simulink model "Citation"  (Simulink 10.1)
settings: Solver=ode5  StartTime=0.0  StopTime=100  FixedStep=0.01  RelTol=1e-3  EnableMultiTasking=on
values from neighbouring files (symbols this model uses):
  cv1 = 20000    [gear_params.m]
  cv2 = cv1    (= 20000)    [gear_params.m]
  cv3 = 4000    [gear_params.m]
  cv4 = 20000    [gear_params.m]
  deltagmax1 = 0.25    [gear_params.m]
  deltagmax2 = deltagmax1    (= 0.25)    [gear_params.m]
  deltagmax3 = 0.24    [gear_params.m]
  deltagmax4 = 0.02    [gear_params.m]
  kt1 = 525020    [gear_params.m]
  kt2 = kt1    (= 525020)    [gear_params.m]
  kt3 = 457050    [gear_params.m]
  murol = 0.03*10    (= 0.3)    [gear_params.m]
  P1 = 2000    [gear_params.m]
  P2 = P1    (= 2000)    [gear_params.m]
  P3 = 2550    [gear_params.m]
  P4 = 40000    [gear_params.m]
  x0 = []    [cessnac550_3d_sfnc.m]    (also in sfunxyz.m)
  xl1 = xcg-6.858    [gear_params.m]
  xl2 = xcg-6.858    [gear_params.m]
  xl3 = xcg-2.0752    [gear_params.m]
  xl4 = xcg-12.742    [gear_params.m]
  yl1 = 1.918    [gear_params.m]
  yl2 = -1.918    [gear_params.m]
  yl3 = 0    [gear_params.m]
  yl4 = 0    [gear_params.m]
  zl1 = zcg-1.701    [gear_params.m]
  zl2 = zcg-1.701    [gear_params.m]
  zl3 = zcg-1.7488    [gear_params.m]
  zl4 = zcg-2.78    [gear_params.m]
undefined symbols (not defined in the file or in its folder): chord, Deng, ealphag, ealphas, g0, hDME, hGS, lh, massinit, matbuaf, matdaf, matdam, matdbbf, matdeaf, matdgaf, matdqaf, matduaf, matdwaw, matedhr, mateif, matelhr, matemhr, matemv1, matemv2, matemve, matetam, mateuaf, matfaaf, matfaxl, matff, matibaf, matibmh, matipaf, matipmh, matiraf, matiuaf, matiwaf, matlaf, matlam, matleaf, matleam, matlgaf, matlqaf, matluaf, matmaaf, matmaam, matmaf, matmam, matmbbf, matmeaf, matmeam, matmgaf, matmqaf, matmrbr, matn1d, matn2d, matnbab, matnbaf, matnbmh, matnpaf ... (+49)
undefined symbols (not defined in the file): matibb
libraries: vrlib x1
(part 4 of 4)

== system Citation/Cessna Citation 500/Citation model DASMAT/AIRCRAFT MODEL/AFM/Aeromod/SubSystem/model/CLCAL/CLGEAF ==
  alpha : Inport
  deltaf : Inport  Port=2
  Prod : Product  InputSameDT=on  SaturateOnIntegerOverflow=on  OutDataTypeStr=Inherit: Same as first input
  Sat : Saturate  UpperLimit=0.04  LowerLimit=-inf
  Sum : Sum  InputSameDT=on  SaturateOnIntegerOverflow=on  OutDataTypeStr=Inherit: Same as first input
  VDOMMYR37 : Lookup  InputValues=vdommyr37(1,:)  Table=vdommyr37(2,:)  SaturateOnIntegerOverflow=on
  VDOMMYR40 : Gain  Gain=1.6  SaturateOnIntegerOverflow=on  OutDataTypeStr=Inherit: Same as input  ParamDataTypeStr=Inherit: Same as input
  rad2deg : Gain  Gain=(180/pi)  SaturateOnIntegerOverflow=on  OutDataTypeStr=Inherit: Same as input  ParamDataTypeStr=Inherit: Same as input
  CLGEAF : Outport
  wires:
  VDOMMYR37/1 -> VDOMMYR40/1, Prod/2
  rad2deg/1 -> Prod/1
  Sat/1 -> rad2deg/1
  alpha/1 -> Sat/1
  deltaf/1 -> VDOMMYR37/1
  VDOMMYR40/1 -> Sum/2
  Prod/1 -> Sum/1
  Sum/1 -> CLGEAF/1

== system Citation/Cessna Citation 500/Citation model DASMAT/AIRCRAFT MODEL/AFM/Aeromod/SubSystem/model/CLCAL/SP0 ==
  deltae : Inport
  Abs : Abs  SaturateOnIntegerOverflow=on
  Fcn : Fcn  Expr=(0.087+0.25*(u[1]-0.087))/(u[1]+1e-11)
  Prod : Product  InputSameDT=on  SaturateOnIntegerOverflow=on  OutDataTypeStr=Inherit: Same as first input
  Sat : Saturate  UpperLimit=1  LowerLimit=-inf
  SP0 : Outport
  wires:
  deltae/1 -> Prod/1, Abs/1
  Sat/1 -> Prod/2
  Fcn/1 -> Sat/1
  Abs/1 -> Fcn/1
  Prod/1 -> SP0/1

== system Citation/Cessna Citation 500/Citation model DASMAT/AIRCRAFT MODEL/AFM/Aeromod/SubSystem/model/CLLCAL/CIBAB ==
  note: 02-11-2000
      | Modified by A. R. Veldhuijzen
      | sftable3.m was replaced with table3.dll
      | X and Y are exchanged in this Mathworks implementation
  x0 : Inport
  y0 : Inport  Port=2
  z0 : Inport  Port=3
  Mux : Mux  Inputs=3
  S-function : S-Function  FunctionName=table3  Parameters=yindex, xindex ,zindex, table  SFunctionDeploymentMode=off  EnableBusSupport=off
  out_1 : Outport
  wires:
  z0/1 -> Mux/3
  y0/1 -> Mux/1
  x0/1 -> Mux/2
  Mux/1 -> S-function/1
  S-function/1 -> out_1/1

== system Citation/Cessna Citation 500/Citation model DASMAT/AIRCRAFT MODEL/AFM/Aeromod/SubSystem/model/CLLCAL/LFACT ==
  hcg : Inport
  Sat : Saturate  UpperLimit=1  LowerLimit=0
  hrunway : Fcn  Expr=1-(u[1]-1)/30
  LFACT : Outport
  wires:
  Sat/1 -> LFACT/1
  hcg/1 -> hrunway/1
  hrunway/1 -> Sat/1

== system Citation/Cessna Citation 500/Citation model DASMAT/AIRCRAFT MODEL/AFM/Aeromod/SubSystem/model/CMCAL/EALPHA ==
  alpha : Inport
  deltaf : Inport  Port=2
  Fcn : Fcn  Expr=1-u[1]*u[2]
  Mux : Mux  Inputs=2
  Sat : Saturate  UpperLimit=1  LowerLimit=0
  Sum : Sum  Inputs=+-  InputSameDT=on  SaturateOnIntegerOverflow=on  OutDataTypeStr=Inherit: Same as first input
  ealphag : Lookup  InputValues=ealphag(1,:)  Table=ealphag(2,:)  SaturateOnIntegerOverflow=on
  ealphas : Lookup  InputValues=ealphas(1,:)  Table=ealphas(2,:)  SaturateOnIntegerOverflow=on
  EALPHA : Outport
  wires:
  deltaf/1 -> ealphag/1, ealphas/1
  alpha/1 -> Sum/1
  Mux/1 -> Fcn/1
  ealphag/1 -> Mux/2
  ealphas/1 -> Sum/2
  Sum/1 -> Mux/1
  Fcn/1 -> Sat/1
  Sat/1 -> EALPHA/1

== system Citation/Cessna Citation 500/Citation model DASMAT/AIRCRAFT MODEL/AFM/Aeromod/SubSystem/model/CMCAL/LFCMEGAF ==
  alpha : Inport
  Abs : Abs  SaturateOnIntegerOverflow=on
  Fcn : Fcn  Expr=1-5*u[1]
  Neg : Gain  Gain=-1  SaturateOnIntegerOverflow=on  OutDataTypeStr=Inherit: Same as input  ParamDataTypeStr=Inherit: Same as input
  Sat : Saturate  UpperLimit=inf  LowerLimit=0.25
  LFCMEGAF : Outport
  wires:
  Fcn/1 -> Sat/1
  alpha/1 -> Abs/1
  Abs/1 -> Fcn/1
  Sat/1 -> Neg/1
  Neg/1 -> LFCMEGAF/1

== system Citation/Cessna Citation 500/Citation model DASMAT/AIRCRAFT MODEL/AFM/Aeromod/SubSystem/model/CYCAL/LSFACT ==
  deltar : Inport
  Abs : Abs  SaturateOnIntegerOverflow=on
  Fcn : Fcn  Expr=0.06981/u[1]+2*(u[1]-0.06981)
  Sat : Saturate  UpperLimit=inf  LowerLimit=0.06981
  LSFACT : Outport
  wires:
  deltar/1 -> Abs/1
  Abs/1 -> Sat/1
  Sat/1 -> Fcn/1
  Fcn/1 -> LSFACT/1

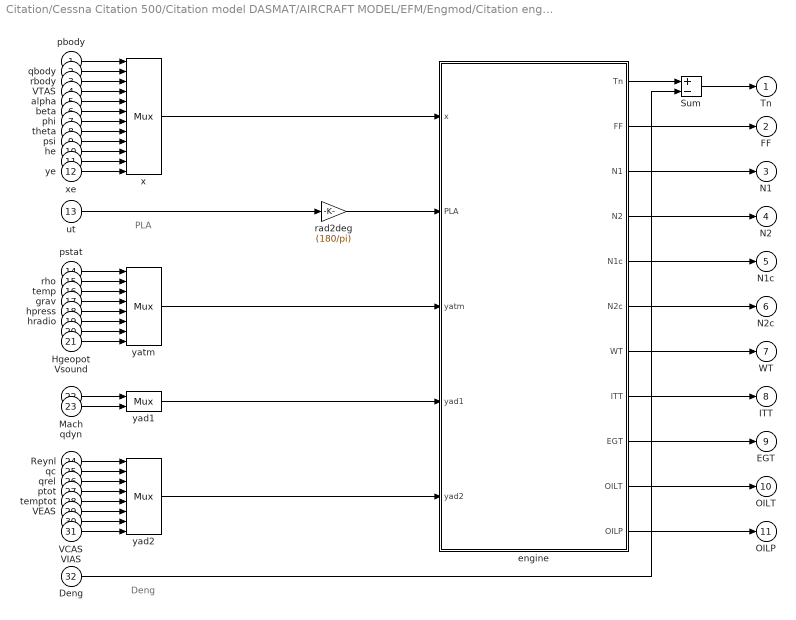
== system Citation/Cessna Citation 500/Citation model DASMAT/AIRCRAFT MODEL/EFM/Engmod/Citation eng_mod/Subsystem1/JT15 Dynamic/Subsystem ==
  note: Deng
  note: PLA
  pbody : Inport
  qbody : Inport  Port=2
  rbody : Inport  Port=3
  VTAS : Inport  Port=4
  alpha : Inport  Port=5
  beta : Inport  Port=6
  phi : Inport  Port=7
  theta : Inport  Port=8
  psi : Inport  Port=9
  he : Inport  Port=10
  xe : Inport  Port=11
  ye : Inport  Port=12
  ut : Inport  Port=13
  pstat : Inport  Port=14
  rho : Inport  Port=15
  temp : Inport  Port=16
  grav : Inport  Port=17
  hpress : Inport  Port=18
  hradio : Inport  Port=19
  Hgeopot : Inport  Port=20
  Vsound : Inport  Port=21
  Mach : Inport  Port=22
  qdyn : Inport  Port=23
  Reynl : Inport  Port=24
  qc : Inport  Port=25
  qrel : Inport  Port=26
  ptot : Inport  Port=27
  temptot : Inport  Port=28
  VEAS : Inport  Port=29
  VCAS : Inport  Port=30
  VIAS : Inport  Port=31
  Deng : Inport  Port=32
  Sum : Sum  Inputs=+-  InputSameDT=on  SaturateOnIntegerOverflow=on  OutDataTypeStr=Inherit: Same as first input
  engine : Subsystem
  rad2deg : Gain  Gain=(180/pi)  SaturateOnIntegerOverflow=on  OutDataTypeStr=Inherit: Same as input  ParamDataTypeStr=Inherit: Same as input
  x : Mux  Inputs=12
  yad1 : Mux  Inputs=2
  yad2 : Mux  Inputs=8
  yatm : Mux  Inputs=8
  Tn : Outport
  FF : Outport  Port=2
  N1 : Outport  Port=3
  N2 : Outport  Port=4
  N1c : Outport  Port=5
  N2c : Outport  Port=6
  WT : Outport  Port=7
  ITT : Outport  Port=8
  EGT : Outport  Port=9
  OILT : Outport  Port=10
  OILP : Outport  Port=11
  wires:
  Deng/1 -> Sum/2
  engine/1(Tn) -> Sum/1
  Sum/1 -> Tn/1
  Vsound/1 -> yatm/8
  engine/11(OILP) -> OILP/1
  engine/10(OILT) -> OILT/1
  rad2deg/1 -> engine/2(PLA)
  ut/1 -> rad2deg/1
  engine/9(EGT) -> EGT/1
  engine/8(ITT) -> ITT/1
  engine/7(WT) -> WT/1
  engine/6(N2c) -> N2c/1
  engine/5(N1c) -> N1c/1
  engine/4(N2) -> N2/1
  engine/3(N1) -> N1/1
  engine/2(FF) -> FF/1
  yad1/1 -> engine/4(yad1)
  yatm/1 -> engine/3(yatm)
  yad2/1 -> engine/5(yad2)
  qdyn/1 -> yad1/2
  Mach/1 -> yad1/1
  Reynl/1 -> yad2/1
  qc/1 -> yad2/2
  VCAS/1 -> yad2/7
  temptot/1 -> yad2/5
  qrel/1 -> yad2/3
  VIAS/1 -> yad2/8
  VEAS/1 -> yad2/6
  ptot/1 -> yad2/4
  ye/1 -> x/12
  xe/1 -> x/11
  he/1 -> x/10
  psi/1 -> x/9
  VTAS/1 -> x/4
  beta/1 -> x/6
  theta/1 -> x/8
  rbody/1 -> x/3
  alpha/1 -> x/5
  phi/1 -> x/7
  qbody/1 -> x/2
  pbody/1 -> x/1
  pstat/1 -> yatm/1
  rho/1 -> yatm/2
  Hgeopot/1 -> yatm/7
  hpress/1 -> yatm/5
  temp/1 -> yatm/3
  hradio/1 -> yatm/6
  grav/1 -> yatm/4
  x/1 -> engine/1(x)

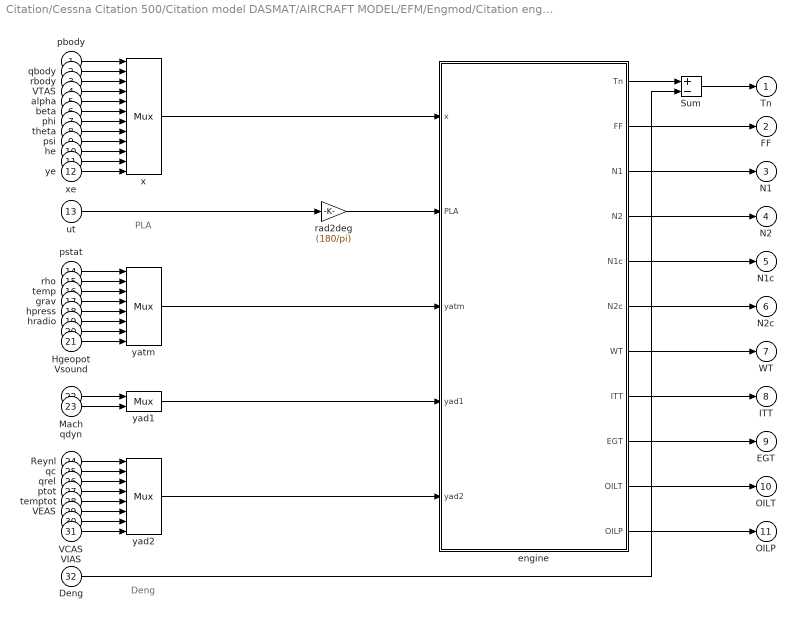
== system Citation/Cessna Citation 500/Citation model DASMAT/AIRCRAFT MODEL/EFM/Engmod/Citation eng_mod/Subsystem1/JT15 Dynamic1/Subsystem ==
  note: Deng
  note: PLA
  pbody : Inport
  qbody : Inport  Port=2
  rbody : Inport  Port=3
  VTAS : Inport  Port=4
  alpha : Inport  Port=5
  beta : Inport  Port=6
  phi : Inport  Port=7
  theta : Inport  Port=8
  psi : Inport  Port=9
  he : Inport  Port=10
  xe : Inport  Port=11
  ye : Inport  Port=12
  ut : Inport  Port=13
  pstat : Inport  Port=14
  rho : Inport  Port=15
  temp : Inport  Port=16
  grav : Inport  Port=17
  hpress : Inport  Port=18
  hradio : Inport  Port=19
  Hgeopot : Inport  Port=20
  Vsound : Inport  Port=21
  Mach : Inport  Port=22
  qdyn : Inport  Port=23
  Reynl : Inport  Port=24
  qc : Inport  Port=25
  qrel : Inport  Port=26
  ptot : Inport  Port=27
  temptot : Inport  Port=28
  VEAS : Inport  Port=29
  VCAS : Inport  Port=30
  VIAS : Inport  Port=31
  Deng : Inport  Port=32
  Sum : Sum  Inputs=+-  InputSameDT=on  SaturateOnIntegerOverflow=on  OutDataTypeStr=Inherit: Same as first input
  engine : Subsystem
  rad2deg : Gain  Gain=(180/pi)  SaturateOnIntegerOverflow=on  OutDataTypeStr=Inherit: Same as input  ParamDataTypeStr=Inherit: Same as input
  x : Mux  Inputs=12
  yad1 : Mux  Inputs=2
  yad2 : Mux  Inputs=8
  yatm : Mux  Inputs=8
  Tn : Outport
  FF : Outport  Port=2
  N1 : Outport  Port=3
  N2 : Outport  Port=4
  N1c : Outport  Port=5
  N2c : Outport  Port=6
  WT : Outport  Port=7
  ITT : Outport  Port=8
  EGT : Outport  Port=9
  OILT : Outport  Port=10
  OILP : Outport  Port=11
  wires:
  Deng/1 -> Sum/2
  engine/1(Tn) -> Sum/1
  Sum/1 -> Tn/1
  Vsound/1 -> yatm/8
  engine/11(OILP) -> OILP/1
  engine/10(OILT) -> OILT/1
  rad2deg/1 -> engine/2(PLA)
  ut/1 -> rad2deg/1
  engine/9(EGT) -> EGT/1
  engine/8(ITT) -> ITT/1
  engine/7(WT) -> WT/1
  engine/6(N2c) -> N2c/1
  engine/5(N1c) -> N1c/1
  engine/4(N2) -> N2/1
  engine/3(N1) -> N1/1
  engine/2(FF) -> FF/1
  yad1/1 -> engine/4(yad1)
  yatm/1 -> engine/3(yatm)
  yad2/1 -> engine/5(yad2)
  qdyn/1 -> yad1/2
  Mach/1 -> yad1/1
  Reynl/1 -> yad2/1
  qc/1 -> yad2/2
  VCAS/1 -> yad2/7
  temptot/1 -> yad2/5
  qrel/1 -> yad2/3
  VIAS/1 -> yad2/8
  VEAS/1 -> yad2/6
  ptot/1 -> yad2/4
  ye/1 -> x/12
  xe/1 -> x/11
  he/1 -> x/10
  psi/1 -> x/9
  VTAS/1 -> x/4
  beta/1 -> x/6
  theta/1 -> x/8
  rbody/1 -> x/3
  alpha/1 -> x/5
  phi/1 -> x/7
  qbody/1 -> x/2
  pbody/1 -> x/1
  pstat/1 -> yatm/1
  rho/1 -> yatm/2
  Hgeopot/1 -> yatm/7
  hpress/1 -> yatm/5
  temp/1 -> yatm/3
  hradio/1 -> yatm/6
  grav/1 -> yatm/4
  x/1 -> engine/1(x)

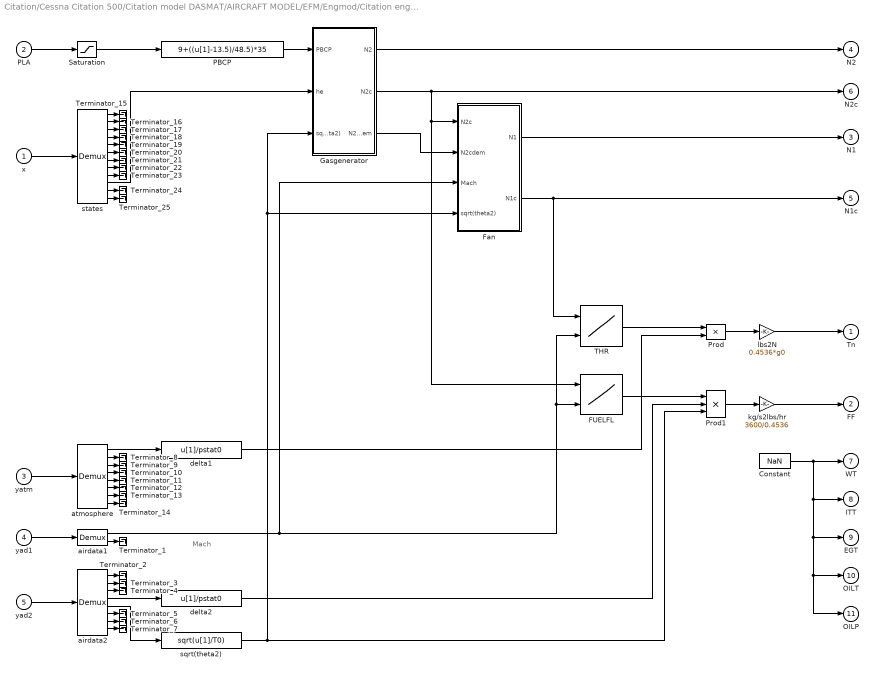
== system Citation/Cessna Citation 500/Citation model DASMAT/AIRCRAFT MODEL/EFM/Engmod/Citation eng_mod/Subsystem1/JT15 Dynamic/Subsystem/engine ==
  note: Mach
  x : Inport
  PLA : Inport  Port=2
  yatm : Inport  Port=3
  yad1 : Inport  Port=4
  yad2 : Inport  Port=5
  Constant : Constant  Value=NaN
  FUELFL : Lookup2D  RowIndex=matff(2:14,1)  ColumnIndex=matff(1,2:14)  Table=matff(2:14,2:14)  SaturateOnIntegerOverflow=on  InputSameDT=on
  Fan : Subsystem
  Gasgenerator : Subsystem
  PBCP : Fcn  Expr=9+((u[1]-13.5)/48.5)*35
  Prod : Product  InputSameDT=on  SaturateOnIntegerOverflow=on  OutDataTypeStr=Inherit: Same as first input
  Prod1 : Product  Inputs=3  InputSameDT=on  SaturateOnIntegerOverflow=on  OutDataTypeStr=Inherit: Same as first input
  Saturation : Saturate  UpperLimit=62  LowerLimit=13.5
  THR : Lookup2D  RowIndex=matthr(2:12,1)  ColumnIndex=matthr(1,2:12)  Table=matthr(2:12,2:12)  SaturateOnIntegerOverflow=on  InputSameDT=on
  Terminator_{1..25} (25 alike) : Terminator
  airdata1 : Demux  Outputs=2
      settings: DisplayOption=none
  airdata2 : Demux  Outputs=8
      settings: DisplayOption=none
  atmosphere : Demux  Outputs=8
      settings: DisplayOption=none
  delta1 : Fcn  Expr=u[1]/pstat0
  delta2 : Fcn  Expr=u[1]/pstat0
  kg/s2lbs/hr : Gain  Gain=3600/0.4536  SaturateOnIntegerOverflow=on  OutDataTypeStr=Inherit: Same as input  ParamDataTypeStr=Inherit: Same as input
  lbs2N : Gain  Gain=0.4536*g0  SaturateOnIntegerOverflow=on  OutDataTypeStr=Inherit: Same as input  ParamDataTypeStr=Inherit: Same as input
  sqrt(theta2) : Fcn  Expr=sqrt(u[1]/T0)
  states : Demux  Outputs=12
      settings: DisplayOption=none
  Tn : Outport
  FF : Outport  Port=2
  N1 : Outport  Port=3
  N2 : Outport  Port=4
  N1c : Outport  Port=5
  N2c : Outport  Port=6
  WT : Outport  Port=7
  ITT : Outport  Port=8
  EGT : Outport  Port=9
  OILT : Outport  Port=10
  OILP : Outport  Port=11
  wires:
  states/12 -> Terminator_25/1
  states/11 -> Terminator_24/1
  states/9 -> Terminator_23/1
  states/8 -> Terminator_22/1
  states/7 -> Terminator_21/1
  states/6 -> Terminator_20/1
  states/5 -> Terminator_19/1
  states/4 -> Terminator_18/1
  states/3 -> Terminator_17/1
  states/2 -> Terminator_16/1
  states/1 -> Terminator_15/1
  atmosphere/8 -> Terminator_14/1
  atmosphere/7 -> Terminator_13/1
  atmosphere/6 -> Terminator_12/1
  atmosphere/5 -> Terminator_11/1
  atmosphere/4 -> Terminator_10/1
  atmosphere/3 -> Terminator_9/1
  atmosphere/2 -> Terminator_8/1
  airdata2/8 -> Terminator_7/1
  airdata2/7 -> Terminator_6/1
  airdata2/6 -> Terminator_5/1
  airdata2/3 -> Terminator_4/1
  airdata2/2 -> Terminator_3/1
  airdata2/1 -> Terminator_2/1
  airdata1/2 -> Terminator_1/1
  Fan/2(N1c) -> THR/1, N1c/1
  Gasgenerator/2(N2c) -> Fan/1(N2c), FUELFL/1, N2c/1
  Gasgenerator/3(N2cdem) -> Fan/2(N2cdem)
  airdata1/1 -> Fan/3(Mach), FUELFL/2, THR/2
  Fan/1(N1) -> N1/1
  sqrt(theta2)/1 -> Fan/4(sqrt(theta2)), Gasgenerator/3(sqrt(theta2)), Prod1/3
  yad2/1 -> airdata2/1
  yad1/1 -> airdata1/1
  yatm/1 -> atmosphere/1
  airdata2/4 -> delta2/1
  airdata2/5 -> sqrt(theta2)/1
  Constant/1 -> ITT/1, EGT/1, OILT/1, OILP/1, WT/1
  Gasgenerator/1(N2) -> N2/1
  delta1/1 -> Prod/2
  Prod/1 -> lbs2N/1
  THR/1 -> Prod/1
  lbs2N/1 -> Tn/1
  states/10 -> Gasgenerator/2(he)
  delta2/1 -> Prod1/2
  atmosphere/1 -> delta1/1
  Prod1/1 -> kg/s2lbs/hr/1
  kg/s2lbs/hr/1 -> FF/1
  Saturation/1 -> PBCP/1
  PLA/1 -> Saturation/1
  x/1 -> states/1
  PBCP/1 -> Gasgenerator/1(PBCP)
  FUELFL/1 -> Prod1/1

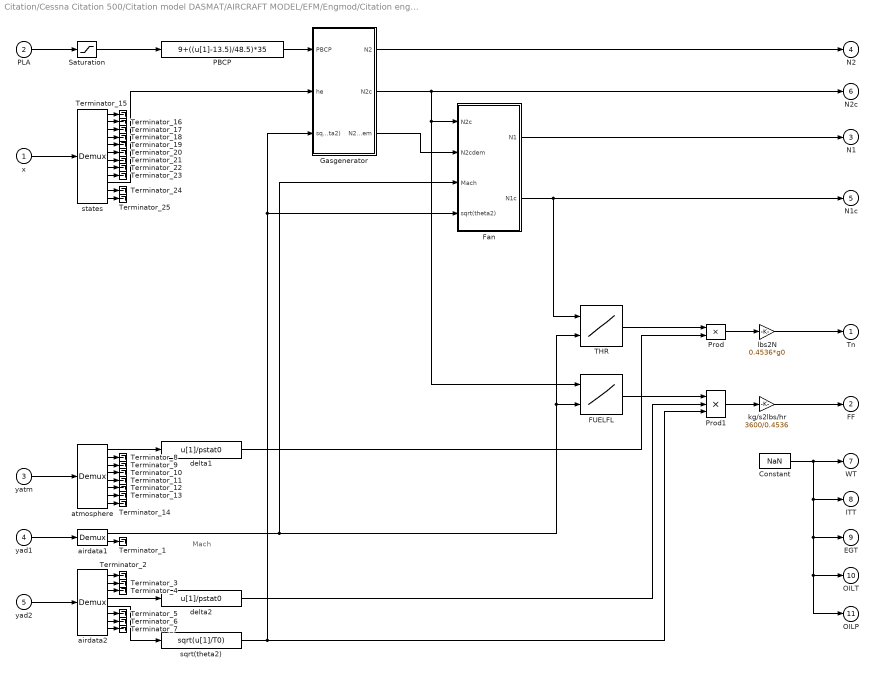
== system Citation/Cessna Citation 500/Citation model DASMAT/AIRCRAFT MODEL/EFM/Engmod/Citation eng_mod/Subsystem1/JT15 Dynamic1/Subsystem/engine ==
  note: Mach
  x : Inport
  PLA : Inport  Port=2
  yatm : Inport  Port=3
  yad1 : Inport  Port=4
  yad2 : Inport  Port=5
  Constant : Constant  Value=NaN
  FUELFL : Lookup2D  RowIndex=matff(2:14,1)  ColumnIndex=matff(1,2:14)  Table=matff(2:14,2:14)  SaturateOnIntegerOverflow=on  InputSameDT=on
  Fan : Subsystem
  Gasgenerator : Subsystem
  PBCP : Fcn  Expr=9+((u[1]-13.5)/48.5)*35
  Prod : Product  InputSameDT=on  SaturateOnIntegerOverflow=on  OutDataTypeStr=Inherit: Same as first input
  Prod1 : Product  Inputs=3  InputSameDT=on  SaturateOnIntegerOverflow=on  OutDataTypeStr=Inherit: Same as first input
  Saturation : Saturate  UpperLimit=62  LowerLimit=13.5
  THR : Lookup2D  RowIndex=matthr(2:12,1)  ColumnIndex=matthr(1,2:12)  Table=matthr(2:12,2:12)  SaturateOnIntegerOverflow=on  InputSameDT=on
  Terminator_{1..25} (25 alike) : Terminator
  airdata1 : Demux  Outputs=2
      settings: DisplayOption=none
  airdata2 : Demux  Outputs=8
      settings: DisplayOption=none
  atmosphere : Demux  Outputs=8
      settings: DisplayOption=none
  delta1 : Fcn  Expr=u[1]/pstat0
  delta2 : Fcn  Expr=u[1]/pstat0
  kg/s2lbs/hr : Gain  Gain=3600/0.4536  SaturateOnIntegerOverflow=on  OutDataTypeStr=Inherit: Same as input  ParamDataTypeStr=Inherit: Same as input
  lbs2N : Gain  Gain=0.4536*g0  SaturateOnIntegerOverflow=on  OutDataTypeStr=Inherit: Same as input  ParamDataTypeStr=Inherit: Same as input
  sqrt(theta2) : Fcn  Expr=sqrt(u[1]/T0)
  states : Demux  Outputs=12
      settings: DisplayOption=none
  Tn : Outport
  FF : Outport  Port=2
  N1 : Outport  Port=3
  N2 : Outport  Port=4
  N1c : Outport  Port=5
  N2c : Outport  Port=6
  WT : Outport  Port=7
  ITT : Outport  Port=8
  EGT : Outport  Port=9
  OILT : Outport  Port=10
  OILP : Outport  Port=11
  wires:
  states/12 -> Terminator_25/1
  states/11 -> Terminator_24/1
  states/9 -> Terminator_23/1
  states/8 -> Terminator_22/1
  states/7 -> Terminator_21/1
  states/6 -> Terminator_20/1
  states/5 -> Terminator_19/1
  states/4 -> Terminator_18/1
  states/3 -> Terminator_17/1
  states/2 -> Terminator_16/1
  states/1 -> Terminator_15/1
  atmosphere/8 -> Terminator_14/1
  atmosphere/7 -> Terminator_13/1
  atmosphere/6 -> Terminator_12/1
  atmosphere/5 -> Terminator_11/1
  atmosphere/4 -> Terminator_10/1
  atmosphere/3 -> Terminator_9/1
  atmosphere/2 -> Terminator_8/1
  airdata2/8 -> Terminator_7/1
  airdata2/7 -> Terminator_6/1
  airdata2/6 -> Terminator_5/1
  airdata2/3 -> Terminator_4/1
  airdata2/2 -> Terminator_3/1
  airdata2/1 -> Terminator_2/1
  airdata1/2 -> Terminator_1/1
  Fan/2(N1c) -> THR/1, N1c/1
  Gasgenerator/2(N2c) -> Fan/1(N2c), FUELFL/1, N2c/1
  Gasgenerator/3(N2cdem) -> Fan/2(N2cdem)
  airdata1/1 -> Fan/3(Mach), FUELFL/2, THR/2
  Fan/1(N1) -> N1/1
  sqrt(theta2)/1 -> Fan/4(sqrt(theta2)), Gasgenerator/3(sqrt(theta2)), Prod1/3
  yad2/1 -> airdata2/1
  yad1/1 -> airdata1/1
  yatm/1 -> atmosphere/1
  airdata2/4 -> delta2/1
  airdata2/5 -> sqrt(theta2)/1
  Constant/1 -> ITT/1, EGT/1, OILT/1, OILP/1, WT/1
  Gasgenerator/1(N2) -> N2/1
  delta1/1 -> Prod/2
  Prod/1 -> lbs2N/1
  THR/1 -> Prod/1
  lbs2N/1 -> Tn/1
  states/10 -> Gasgenerator/2(he)
  delta2/1 -> Prod1/2
  atmosphere/1 -> delta1/1
  Prod1/1 -> kg/s2lbs/hr/1
  kg/s2lbs/hr/1 -> FF/1
  Saturation/1 -> PBCP/1
  PLA/1 -> Saturation/1
  x/1 -> states/1
  PBCP/1 -> Gasgenerator/1(PBCP)
  FUELFL/1 -> Prod1/1

== system Citation/Cessna Citation 500/Citation model DASMAT/AIRCRAFT MODEL/EFM/Engmod/Citation eng_mod/Subsystem1/JT15 Dynamic/Subsystem/engine/Fan ==
  note: N1c feedback
  note: N1cdot
  N2c : Inport
  N2cdem : Inport  Port=2
  Mach : Inport  Port=3
  sqrt(theta2) : Inport  Port=4
  Droop : Gain  Gain=2  SaturateOnIntegerOverflow=on  OutDataTypeStr=Inherit: Same as input  ParamDataTypeStr=Inherit: Same as input
  Max accel : Subsystem  mask(Min Value){}
      mask help:
      | Output is minimum value of inputs.
      | y=min(u1,u2)
      mask Help: The Min block produces as output the minimum value of two scalars or vectors. If the inputs are vectors, the output will be a vector containing the minimum elements of the vectors.
      mask Display: disp('Min')
  Max decel : Subsystem  mask(Max Value){}
      mask help:
      | Output is maximum value of inputs.
      | y=max(u1,u2)
      mask Help: The Max block produces as output the maximum value of two scalars or vectors. If the inputs are vectors, the output will be a vector containing the maximum elements of the vectors.
      mask Display: disp('Max')
  N1 state : Integrator  InitialCondition=xt0(2)
  N1D : Lookup2D  RowIndex=matn1d(2:14,1)  ColumnIndex=matn1d(1,2:14)  Table=matn1d(2:14,2:14)  SaturateOnIntegerOverflow=on  InputSameDT=on
  Prod : Product  InputSameDT=on  SaturateOnIntegerOverflow=on  OutDataTypeStr=Inherit: Same as first input
  Sum : Sum  Inputs=+-  InputSameDT=on  SaturateOnIntegerOverflow=on  OutDataTypeStr=Inherit: Same as first input
  fN1cmax : Lookup  InputValues="[0 25 40 70 94  120]"  Table="[0   0   1   12 14  18]"  SaturateOnIntegerOverflow=on
  fN1cmin : Lookup  InputValues="[25     50   60   94 100]"  Table="[-0.05  -0.05    -1    -30 -28]"  SaturateOnIntegerOverflow=on
  N1 : Outport
  N1c : Outport  Port=2
  wires:
  sqrt(theta2)/1 -> Prod/2
  N1 state/1 -> Prod/1, Sum/2, N1c/1
  N2c/1 -> fN1cmin/1, fN1cmax/1
  Max decel/1(out_1) -> N1 state/1
  N1D/1 -> Sum/1
  Max accel/1(out_1) -> Max decel/1(in_1)
  fN1cmax/1 -> Max accel/2(in_2)
  fN1cmin/1 -> Max decel/2(in_2)
  Sum/1 -> Droop/1
  Droop/1 -> Max accel/1(in_1)
  Mach/1 -> N1D/2
  Prod/1 -> N1/1
  N2cdem/1 -> N1D/1

== system Citation/Cessna Citation 500/Citation model DASMAT/AIRCRAFT MODEL/EFM/Engmod/Citation eng_mod/Subsystem1/JT15 Dynamic/Subsystem/engine/Gasgenerator ==
  note: N2 feedback
  note: N2dot
  PBCP : Inport
  he : Inport  Port=2
  sqrt(theta2) : Inport  Port=3
  Droop : Lookup  InputValues=[0 100]  Table="[0.1  2]"  SaturateOnIntegerOverflow=on
  Fcn : Fcn  Expr=u[1]/u[2]
  Fcn1 : Fcn  Expr=u[1]/u[2]
  Governor : Product  InputSameDT=on  SaturateOnIntegerOverflow=on  OutDataTypeStr=Inherit: Same as first input
  Max accel : Subsystem  mask(Max Value){}
      mask help:
      | Output is maximum value of inputs.
      | y=max(u1,u2)
      mask Help: The Max block produces as output the maximum value of two scalars or vectors. If the inputs are vectors, the output will be a vector containing the maximum elements of the vectors.
      mask Display: disp('Max')
  Min accel : Subsystem  mask(Min Value){}
      mask help:
      | Output is minimum value of inputs.
      | y=min(u1,u2)
      mask Help: The Min block produces as output the minimum value of two scalars or vectors. If the inputs are vectors, the output will be a vector containing the minimum elements of the vectors.
      mask Display: disp('Min')
  Mux : Mux  Inputs=2
  Mux1 : Mux  Inputs=2
  N2 state : Integrator  InitialCondition=xt0(1)
  N2D : Lookup2D  RowIndex=matn2d(2:10,1)  ColumnIndex=matn2d(1,2:10)  Table=matn2d(2:10,2:10)  SaturateOnIntegerOverflow=on  InputSameDT=on
  Sum : Sum  Inputs=+-  InputSameDT=on  SaturateOnIntegerOverflow=on  OutDataTypeStr=Inherit: Same as first input
  fN2max : Lookup  InputValues=[25 40 70 94]  Table=[0 3 8 10]  SaturateOnIntegerOverflow=on
  fN2min : Lookup  InputValues="[25     50   60   94 100]"  Table="[-0.05  -0.05    -2    -20 -28]"  SaturateOnIntegerOverflow=on
  ft2FL : Gain  Gain=.01  SaturateOnIntegerOverflow=on  OutDataTypeStr=Inherit: Same as input  ParamDataTypeStr=Inherit: Same as input
  m2ft : Gain  Gain=(1/0.3048)  SaturateOnIntegerOverflow=on  OutDataTypeStr=Inherit: Same as input  ParamDataTypeStr=Inherit: Same as input
  N2 : Outport
  N2c : Outport  Port=2
  N2cdem : Outport  Port=3
  wires:
  sqrt(theta2)/1 -> Mux1/2, Mux/2
  N2D/1 -> Mux/1, Droop/1, Sum/1
  Fcn1/1 -> N2c/1
  Fcn/1 -> N2cdem/1
  Mux1/1 -> Fcn1/1
  Mux/1 -> Fcn/1
  Min accel/1(out_1) -> Max accel/1(in_1)
  ft2FL/1 -> N2D/2
  m2ft/1 -> ft2FL/1
  he/1 -> m2ft/1
  N2 state/1 -> Mux1/1, fN2min/1, fN2max/1, Sum/2, N2/1
  fN2max/1 -> Min accel/2(in_2)
  fN2min/1 -> Max accel/2(in_2)
  PBCP/1 -> N2D/1
  Droop/1 -> Governor/1
  Sum/1 -> Governor/2
  Governor/1 -> Min accel/1(in_1)
  Max accel/1(out_1) -> N2 state/1

== system Citation/Cessna Citation 500/Citation model DASMAT/AIRCRAFT MODEL/EFM/Engmod/Citation eng_mod/Subsystem1/JT15 Dynamic1/Subsystem/engine/Fan ==
  note: N1c feedback
  note: N1cdot
  N2c : Inport
  N2cdem : Inport  Port=2
  Mach : Inport  Port=3
  sqrt(theta2) : Inport  Port=4
  Droop : Gain  Gain=2  SaturateOnIntegerOverflow=on  OutDataTypeStr=Inherit: Same as input  ParamDataTypeStr=Inherit: Same as input
  Max accel : Subsystem  mask(Min Value){}
      mask help:
      | Output is minimum value of inputs.
      | y=min(u1,u2)
      mask Help: The Min block produces as output the minimum value of two scalars or vectors. If the inputs are vectors, the output will be a vector containing the minimum elements of the vectors.
      mask Display: disp('Min')
  Max decel : Subsystem  mask(Max Value){}
      mask help:
      | Output is maximum value of inputs.
      | y=max(u1,u2)
      mask Help: The Max block produces as output the maximum value of two scalars or vectors. If the inputs are vectors, the output will be a vector containing the maximum elements of the vectors.
      mask Display: disp('Max')
  N1 state : Integrator  InitialCondition=xt0(2)
  N1D : Lookup2D  RowIndex=matn1d(2:14,1)  ColumnIndex=matn1d(1,2:14)  Table=matn1d(2:14,2:14)  SaturateOnIntegerOverflow=on  InputSameDT=on
  Prod : Product  InputSameDT=on  SaturateOnIntegerOverflow=on  OutDataTypeStr=Inherit: Same as first input
  Sum : Sum  Inputs=+-  InputSameDT=on  SaturateOnIntegerOverflow=on  OutDataTypeStr=Inherit: Same as first input
  fN1cmax : Lookup  InputValues="[0 25 40 70 94  120]"  Table="[0   0   1   12 14  18]"  SaturateOnIntegerOverflow=on
  fN1cmin : Lookup  InputValues="[25     50   60   94 100]"  Table="[-0.05  -0.05    -1    -30 -28]"  SaturateOnIntegerOverflow=on
  N1 : Outport
  N1c : Outport  Port=2
  wires:
  sqrt(theta2)/1 -> Prod/2
  N1 state/1 -> Prod/1, Sum/2, N1c/1
  N2c/1 -> fN1cmin/1, fN1cmax/1
  Max decel/1(out_1) -> N1 state/1
  N1D/1 -> Sum/1
  Max accel/1(out_1) -> Max decel/1(in_1)
  fN1cmax/1 -> Max accel/2(in_2)
  fN1cmin/1 -> Max decel/2(in_2)
  Sum/1 -> Droop/1
  Droop/1 -> Max accel/1(in_1)
  Mach/1 -> N1D/2
  Prod/1 -> N1/1
  N2cdem/1 -> N1D/1

== system Citation/Cessna Citation 500/Citation model DASMAT/AIRCRAFT MODEL/EFM/Engmod/Citation eng_mod/Subsystem1/JT15 Dynamic1/Subsystem/engine/Gasgenerator ==
  note: N2 feedback
  note: N2dot
  PBCP : Inport
  he : Inport  Port=2
  sqrt(theta2) : Inport  Port=3
  Droop : Lookup  InputValues=[0 100]  Table="[0.1  2]"  SaturateOnIntegerOverflow=on
  Fcn : Fcn  Expr=u[1]/u[2]
  Fcn1 : Fcn  Expr=u[1]/u[2]
  Governor : Product  InputSameDT=on  SaturateOnIntegerOverflow=on  OutDataTypeStr=Inherit: Same as first input
  Max accel : Subsystem  mask(Max Value){}
      mask help:
      | Output is maximum value of inputs.
      | y=max(u1,u2)
      mask Help: The Max block produces as output the maximum value of two scalars or vectors. If the inputs are vectors, the output will be a vector containing the maximum elements of the vectors.
      mask Display: disp('Max')
  Min accel : Subsystem  mask(Min Value){}
      mask help:
      | Output is minimum value of inputs.
      | y=min(u1,u2)
      mask Help: The Min block produces as output the minimum value of two scalars or vectors. If the inputs are vectors, the output will be a vector containing the minimum elements of the vectors.
      mask Display: disp('Min')
  Mux : Mux  Inputs=2
  Mux1 : Mux  Inputs=2
  N2 state : Integrator  InitialCondition=xt0(1)
  N2D : Lookup2D  RowIndex=matn2d(2:10,1)  ColumnIndex=matn2d(1,2:10)  Table=matn2d(2:10,2:10)  SaturateOnIntegerOverflow=on  InputSameDT=on
  Sum : Sum  Inputs=+-  InputSameDT=on  SaturateOnIntegerOverflow=on  OutDataTypeStr=Inherit: Same as first input
  fN2max : Lookup  InputValues=[25 40 70 94]  Table=[0 3 8 10]  SaturateOnIntegerOverflow=on
  fN2min : Lookup  InputValues="[25     50   60   94 100]"  Table="[-0.05  -0.05    -2    -20 -28]"  SaturateOnIntegerOverflow=on
  ft2FL : Gain  Gain=.01  SaturateOnIntegerOverflow=on  OutDataTypeStr=Inherit: Same as input  ParamDataTypeStr=Inherit: Same as input
  m2ft : Gain  Gain=(1/0.3048)  SaturateOnIntegerOverflow=on  OutDataTypeStr=Inherit: Same as input  ParamDataTypeStr=Inherit: Same as input
  N2 : Outport
  N2c : Outport  Port=2
  N2cdem : Outport  Port=3
  wires:
  sqrt(theta2)/1 -> Mux1/2, Mux/2
  N2D/1 -> Mux/1, Droop/1, Sum/1
  Fcn1/1 -> N2c/1
  Fcn/1 -> N2cdem/1
  Mux1/1 -> Fcn1/1
  Mux/1 -> Fcn/1
  Min accel/1(out_1) -> Max accel/1(in_1)
  ft2FL/1 -> N2D/2
  m2ft/1 -> ft2FL/1
  he/1 -> m2ft/1
  N2 state/1 -> Mux1/1, fN2min/1, fN2max/1, Sum/2, N2/1
  fN2max/1 -> Min accel/2(in_2)
  fN2min/1 -> Max accel/2(in_2)
  PBCP/1 -> N2D/1
  Droop/1 -> Governor/1
  Sum/1 -> Governor/2
  Governor/1 -> Min accel/1(in_1)
  Max accel/1(out_1) -> N2 state/1

== system Citation/Cessna Citation 500/Citation model DASMAT/AIRCRAFT MODEL/EFM/Engmod/Citation eng_mod/Subsystem1/JT15 Dynamic/Subsystem/engine/Fan/Max accel ==
  in_1 : Inport
  in_2 : Inport  Port=2
  Sum : Sum  Inputs=-+  InputSameDT=on  SaturateOnIntegerOverflow=on  OutDataTypeStr=Inherit: Same as first input
  Switch : Switch  SaturateOnIntegerOverflow=on  InputSameDT=on
  out_1 : Outport
  wires:
  in_1/1 -> Sum/1, Switch/1
  in_2/1 -> Sum/2, Switch/3
  Sum/1 -> Switch/2
  Switch/1 -> out_1/1

== system Citation/Cessna Citation 500/Citation model DASMAT/AIRCRAFT MODEL/EFM/Engmod/Citation eng_mod/Subsystem1/JT15 Dynamic/Subsystem/engine/Fan/Max decel ==
  in_1 : Inport
  in_2 : Inport  Port=2
  Sum : Sum  Inputs=+-  InputSameDT=on  SaturateOnIntegerOverflow=on  OutDataTypeStr=Inherit: Same as first input
  Switch : Switch  SaturateOnIntegerOverflow=on  InputSameDT=on
  out_1 : Outport
  wires:
  Switch/1 -> out_1/1
  Sum/1 -> Switch/2
  in_2/1 -> Sum/2, Switch/3
  in_1/1 -> Sum/1, Switch/1

== system Citation/Cessna Citation 500/Citation model DASMAT/AIRCRAFT MODEL/EFM/Engmod/Citation eng_mod/Subsystem1/JT15 Dynamic/Subsystem/engine/Gasgenerator/Max accel ==
  in_1 : Inport
  in_2 : Inport  Port=2
  Sum : Sum  Inputs=+-  InputSameDT=on  SaturateOnIntegerOverflow=on  OutDataTypeStr=Inherit: Same as first input
  Switch : Switch  SaturateOnIntegerOverflow=on  InputSameDT=on
  out_1 : Outport
  wires:
  Switch/1 -> out_1/1
  Sum/1 -> Switch/2
  in_2/1 -> Sum/2, Switch/3
  in_1/1 -> Sum/1, Switch/1

== system Citation/Cessna Citation 500/Citation model DASMAT/AIRCRAFT MODEL/EFM/Engmod/Citation eng_mod/Subsystem1/JT15 Dynamic/Subsystem/engine/Gasgenerator/Min accel ==
  in_1 : Inport
  in_2 : Inport  Port=2
  Sum : Sum  Inputs=-+  InputSameDT=on  SaturateOnIntegerOverflow=on  OutDataTypeStr=Inherit: Same as first input
  Switch : Switch  SaturateOnIntegerOverflow=on  InputSameDT=on
  out_1 : Outport
  wires:
  in_1/1 -> Sum/1, Switch/1
  in_2/1 -> Sum/2, Switch/3
  Sum/1 -> Switch/2
  Switch/1 -> out_1/1

== system Citation/Cessna Citation 500/Citation model DASMAT/AIRCRAFT MODEL/EFM/Engmod/Citation eng_mod/Subsystem1/JT15 Dynamic1/Subsystem/engine/Fan/Max accel ==
  in_1 : Inport
  in_2 : Inport  Port=2
  Sum : Sum  Inputs=-+  InputSameDT=on  SaturateOnIntegerOverflow=on  OutDataTypeStr=Inherit: Same as first input
  Switch : Switch  SaturateOnIntegerOverflow=on  InputSameDT=on
  out_1 : Outport
  wires:
  in_1/1 -> Sum/1, Switch/1
  in_2/1 -> Sum/2, Switch/3
  Sum/1 -> Switch/2
  Switch/1 -> out_1/1

== system Citation/Cessna Citation 500/Citation model DASMAT/AIRCRAFT MODEL/EFM/Engmod/Citation eng_mod/Subsystem1/JT15 Dynamic1/Subsystem/engine/Fan/Max decel ==
  in_1 : Inport
  in_2 : Inport  Port=2
  Sum : Sum  Inputs=+-  InputSameDT=on  SaturateOnIntegerOverflow=on  OutDataTypeStr=Inherit: Same as first input
  Switch : Switch  SaturateOnIntegerOverflow=on  InputSameDT=on
  out_1 : Outport
  wires:
  Switch/1 -> out_1/1
  Sum/1 -> Switch/2
  in_2/1 -> Sum/2, Switch/3
  in_1/1 -> Sum/1, Switch/1

== system Citation/Cessna Citation 500/Citation model DASMAT/AIRCRAFT MODEL/EFM/Engmod/Citation eng_mod/Subsystem1/JT15 Dynamic1/Subsystem/engine/Gasgenerator/Max accel ==
  in_1 : Inport
  in_2 : Inport  Port=2
  Sum : Sum  Inputs=+-  InputSameDT=on  SaturateOnIntegerOverflow=on  OutDataTypeStr=Inherit: Same as first input
  Switch : Switch  SaturateOnIntegerOverflow=on  InputSameDT=on
  out_1 : Outport
  wires:
  Switch/1 -> out_1/1
  Sum/1 -> Switch/2
  in_2/1 -> Sum/2, Switch/3
  in_1/1 -> Sum/1, Switch/1

== system Citation/Cessna Citation 500/Citation model DASMAT/AIRCRAFT MODEL/EFM/Engmod/Citation eng_mod/Subsystem1/JT15 Dynamic1/Subsystem/engine/Gasgenerator/Min accel ==
  in_1 : Inport
  in_2 : Inport  Port=2
  Sum : Sum  Inputs=-+  InputSameDT=on  SaturateOnIntegerOverflow=on  OutDataTypeStr=Inherit: Same as first input
  Switch : Switch  SaturateOnIntegerOverflow=on  InputSameDT=on
  out_1 : Outport
  wires:
  in_1/1 -> Sum/1, Switch/1
  in_2/1 -> Sum/2, Switch/3
  Sum/1 -> Switch/2
  Switch/1 -> out_1/1

== matlab function MATLAB Function ==
  data: inputs input double; p_est input double; y output double; y_est output double; p_est output double; P output double; P input double
function [y, y_est, p_est, P] = RLS(inputs, p_est, P)

% Initialize aircraft and atmospheric parameters
Ixx = 11187.8;      b = 13.3250;    R        = 287.05;    rho_0    = 1.225;
Iyy = 22854.8;      S = 24.9900;    lam_trop = -0.0065;   h_tropo  = 11;
Izz = 31974.8;      c = 1.9910;     h_0      = 0;         h_strato = 20;
Ixz = 1930.1;       m = 4500;       T_0      = 288.15;    g        = 9.81;

% Initialize state parameters
p       = inputs(1);    he      = inputs(7);    anxb    = inputs(13)*g;
q       = inputs(2);    ye      = inputs(8);    anyb    = inputs(14)*g;
r       = inputs(3);    xe      = inputs(9);    anzb    = inputs(15)*g;
vtas    = inputs(4);    p_dot   = inputs(10);   de      = inputs(16);
alpha   = inputs(5);    q_dot   = inputs(11);   da      = inputs(17);
beta    = inputs(6);    r_dot   = inputs(12);   dr      = inputs(18);

% Calculate atmospheric conditions
rho = rho_0 * (1 + lam_trop*(he/T_0))^(-(g/(R*lam_trop)) - 1);

% Calculate aerydynamic force and moment components
CX = (m*anxb)/(0.5*rho*vtas^2*S);
CY = (m*anyb)/(0.5*rho*vtas^2*S);
CZ = (m*anzb)/(0.5*rho*vtas^2*S);

Cl = (p_dot*Ixx + q*r*(Izz - Iyy) - (p*q + r_dot)*Ixz)/(0.5*rho*vtas^2*S*b);
Cm = (q_dot*Iyy + r*p*(Ixx - Izz) + (p^2 + r^2)*Ixz)/(0.5*rho*vtas^2*S*c);
Cn = (r_dot*Izz + p*q*(Iyy - Ixx) + (q*r + p_dot)*Ixz)/(0.5*rho*vtas^2*S*b);

y1 = CX;
y2 = CY;
y3 = CZ;
y4 = Cl;
y5 = Cm;
y6 = Cn;

% Initialize regression matrix
H_y1 = [1 alpha alpha^2 (q*c/vtas) de 0];
H_y2 = [1 alpha 0 (q*c/vtas) de 0];
H_y3 = [1 alpha 0 (q*c/vtas) de 0];
H_y4 = [1 beta (p*b/2*vtas) (r*b/2*vtas) da dr];
H_y5 = [1 beta (p*b/2*vtas) (r*b/2*vtas) da dr];
H_y6 = [1 beta (p*b/2*vtas) (r*b/2*vtas) da dr];

% Initialize parameter vectors
p_1 = p_est(:,1);
p_2 = p_est(:,2);
p_3 = p_est(:,3);
p_4 = p_est(:,4);
p_5 = p_est(:,5);
p_6 = p_est(:,6);

% Calculate least square gains
L_k1 = P*H_y1' * inv(H_y1*P*H_y1' + 1);
L_k2 = P*H_y2' * inv(H_y2*P*H_y2' + 1);
L_k3 = P*H_y3' * inv(H_y3*P*H_y3' + 1);
L_k4 = P*H_y4' * inv(H_y4*P*H_y4' + 1);
L_k5 = P*H_y5' * inv(H_y5*P*H_y5' + 1);
L_k6 = P*H_y6' * inv(H_y6*P*H_y6' + 1);

% Calculate estimated parameters
p_k1 = p_1 + L_k1*(y1 - H_y1*p_1);
p_k2 = p_2 + L_k2*(y2 - H_y2*p_2);
p_k3 = p_3 + L_k3*(y3 - H_y3*p_3);
p_k4 = p_4 + L_k4*(y4 - H_y4*p_4);
p_k5 = p_5 + L_k5*(y5 - H_y5*p_5);
p_k6 = p_6 + L_k6*(y6 - H_y6*p_6);

% Calculate new covariance
P_k1 = (eye(6) - L_k1*H_y1)*P(:,1);
P_k2 = (eye(6) - L_k2*H_y2)*P(:,2);
P_k3 = (eye(6) - L_k3*H_y3)*P(:,3);
P_k4 = (eye(6) - L_k4*H_y4)*P(:,4);
P_k5 = (eye(6) - L_k5*H_y5)*P(:,5);
P_k6 = (eye(6) - L_k6*H_y6)*P(:,6);

% P_k1 = (eye(6) - L_k1*H_y1)*P;
% P_k2 = (eye(6) - L_k2*H_y2)*P;
% P_k3 = (eye(6) - L_k3*H_y3)*P;
% P_k4 = (eye(6) - L_k4*H_y4)*P;
% P_k5 = (eye(6) - L_k5*H_y5)*P;
% P_k6 = (eye(6) - L_k6*H_y6)*P;

% Update parameters and covariance [COVARIANCE STILL FIGURE OUT]
p_est(:,1) = p_k1;  P(:,1) = P_k1;
p_est(:,2) = p_k2;  P(:,2) = P_k2;
p_est(:,3) = p_k3;  P(:,3) = P_k3;
p_est(:,4) = p_k4;  P(:,4) = P_k4;
p_est(:,5) = p_k5;  P(:,5) = P_k5;
p_est(:,6) = p_k6;  P(:,6) = P_k6;

% p_est(:,1) = p_k1;  P(:,1) = P_k1(:,1);
% p_est(:,2) = p_k2;  P(:,2) = P_k2(:,2);
% p_est(:,3) = p_k3;  P(:,3) = P_k3(:,3);
% p_est(:,4) = p_k4;  P(:,4) = P_k4(:,4);
% p_est(:,5) = p_k5;  P(:,5) = P_k5(:,5);
% p_est(:,6) = p_k6;  P(:,6) = P_k6(:,6);

% Output model
y_est1 = H_y1*p_k1;
y_est2 = H_y2*p_k2;
y_est3 = H_y3*p_k3;
y_est4 = H_y4*p_k4;
y_est5 = H_y5*p_k5;
y_est6 = H_y6*p_k6;

y = [y1,y2,y3,y4,y5,y6];
y_est = [y_est1,y_est2,y_est3,y_est4,y_est5,y_est6];
p_est = p_est;
P = P;
